simulink model "q1"  (R2023a)
settings: Solver=VariableStepAuto  StartTime=0.0  StopTime=10.0  RelTol=1e-3
settings Model: Creator=giri0  LastModifiedBy=giri0

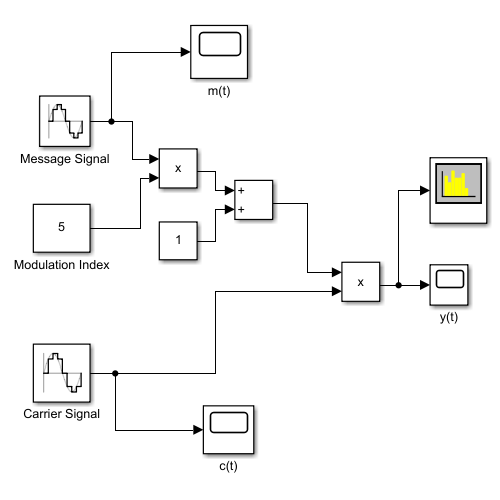
[thumbnail: Simulink's stored preview of the top-level diagram]
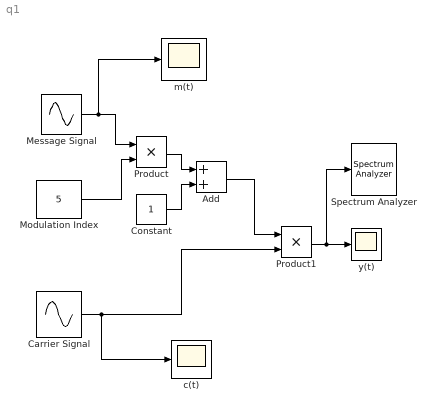
== system q1 ==
  Add : Sum
  Carrier Signal : Sin  Frequency=2*pi*25  SampleTime=1/5000
  Constant : Constant
  Message Signal : Sin  Frequency=2*pi  SampleTime=1/5000
  Modulation Index : Constant  Value=5
  Product : Product
  Product1 : Product
  Spectrum Analyzer : SpectrumAnalyzer  WindowPosition=[512.000000,115.000000,800.000000,500.000000,]  ScopeFrameLocation=window  YLimits=[-118.08875383,52.43550223]  ColorLimits=[-80 20]
  c(t) : Scope
  m(t) : Scope
  y(t) : Scope
  wires:
  Message Signal/1 -> Product/1, m(t)/1
  Modulation Index/1 -> Product/2
  Product/1 -> Add/1
  Constant/1 -> Add/2
  Add/1 -> Product1/1
  Carrier Signal/1 -> c(t)/1, Product1/2
  Product1/1 -> Spectrum Analyzer/1, y(t)/1
